simulink model "rate_limited_systems_controller_design"  (R2021a)
settings: Solver=VariableStepAuto  StartTime=0.0  StopTime=25  RelTol=1e-3
values from neighbouring files (symbols this model uses):
  K_P = 1/abs(freqresp(G_ol,omega_c))    [Anti_windup_example.m]    (also in P_Lead_Lag.m = 1/abs(freqresp(G_ol,omega_c*1i)); Rate_limited_example.m; Rate_limited_exercise.m)
undefined symbols (not defined in the file or in its folder): den_D, den_PI, num_D, num_PI
settings Model: Creator=dimpa  LastModifiedBy=dimpa

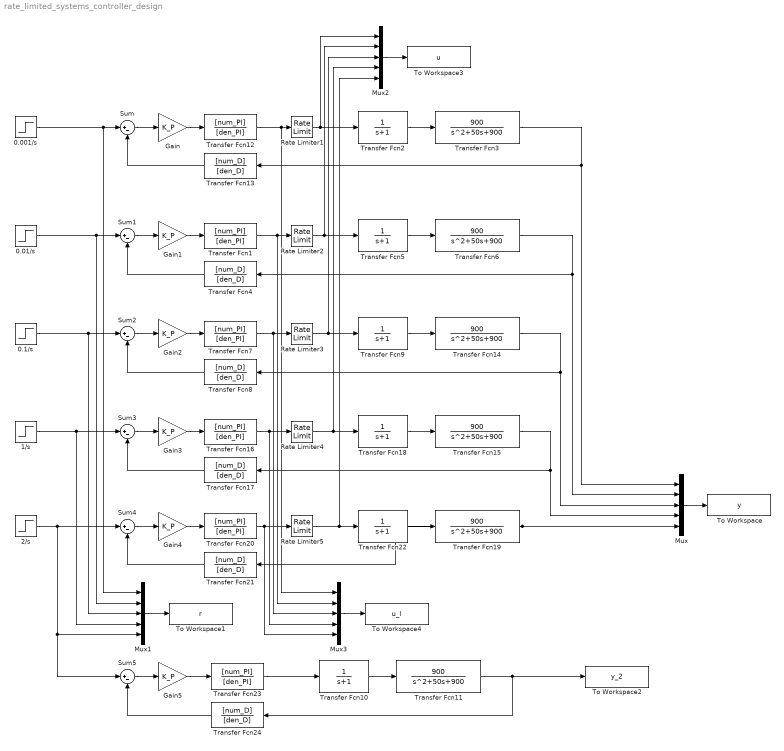
== system rate_limited_systems_controller_design ==
  0.001/s : Step  After=0.001  SampleTime=0
  0.01/s : Step  After=0.01  SampleTime=0
  0.1/s : Step  After=0.1  SampleTime=0
  1/s : Step  SampleTime=0
  2/s : Step  After=2  SampleTime=0
  Gain{,1..5} (6 alike) : Gain  Gain=K_P
  Mux{,1..3} (4 alike) : Mux  Inputs=5
  Rate Limiter{1..5} (5 alike) : RateLimiter  RisingSlewLimit=0.3  SampleTimeMode=inherited
  Sum{,1..5} (6 alike) : Sum  Inputs=|+-
  To Workspace : ToWorkspace  VariableName=y  SaveFormat=Timeseries  SampleTime=-1
  To Workspace1 : ToWorkspace  VariableName=r  SaveFormat=Timeseries  SampleTime=-1
  To Workspace2 : ToWorkspace  VariableName=y_2  SaveFormat=Timeseries  SampleTime=-1
  To Workspace3 : ToWorkspace  VariableName=u  SaveFormat=Timeseries  SampleTime=-1
  To Workspace4 : ToWorkspace  VariableName=u_l  SaveFormat=Timeseries  SampleTime=-1
  Transfer Fcn{1,7,12,16,20,23} (6 alike) : TransferFcn  Numerator=[num_PI]  Denominator=[den_PI]
  Transfer Fcn{2,5,9..10,18,22} (6 alike) : TransferFcn  Denominator=[1 1]
  Transfer Fcn{3,6,11,14..15,19} (6 alike) : TransferFcn  Numerator=[900]  Denominator=[1 50 900]
  Transfer Fcn{4,8,13,17,21,24} (6 alike) : TransferFcn  Numerator=[num_D]  Denominator=[den_D]
  wires:
  0.001/s/1 -> Sum/1, Mux1/1
  0.01/s/1 -> Sum1/1, Mux1/2
  0.1/s/1 -> Sum2/1, Mux1/3
  1/s/1 -> Sum3/1, Mux1/4
  2/s/1 -> Sum4/1, Sum5/1, Mux1/5
  Transfer Fcn19/1 -> Mux/5, Transfer Fcn21/1
  Transfer Fcn2/1 -> Transfer Fcn3/1
  Rate Limiter1/1 -> Transfer Fcn2/1, Mux2/1
  Transfer Fcn15/1 -> Transfer Fcn17/1, Mux/4
  Transfer Fcn14/1 -> Transfer Fcn8/1, Mux/3
  Transfer Fcn6/1 -> Transfer Fcn4/1, Mux/2
  Transfer Fcn3/1 -> Transfer Fcn13/1, Mux/1
  Mux/1 -> To Workspace/1
  Mux1/1 -> To Workspace1/1
  Transfer Fcn10/1 -> Transfer Fcn11/1
  Sum/1 -> Gain/1
  Gain/1 -> Transfer Fcn12/1
  Transfer Fcn12/1 -> Mux3/1, Rate Limiter1/1
  Transfer Fcn13/1 -> Sum/2
  Transfer Fcn4/1 -> Sum1/2
  Transfer Fcn1/1 -> Mux3/2, Rate Limiter2/1
  Gain1/1 -> Transfer Fcn1/1
  Sum1/1 -> Gain1/1
  Rate Limiter2/1 -> Transfer Fcn5/1, Mux2/2
  Transfer Fcn5/1 -> Transfer Fcn6/1
  Transfer Fcn9/1 -> Transfer Fcn14/1
  Rate Limiter3/1 -> Mux2/3, Transfer Fcn9/1
  Sum2/1 -> Gain2/1
  Gain2/1 -> Transfer Fcn7/1
  Transfer Fcn7/1 -> Mux3/3, Rate Limiter3/1
  Transfer Fcn8/1 -> Sum2/2
  Transfer Fcn17/1 -> Sum3/2
  Transfer Fcn16/1 -> Mux3/4, Rate Limiter4/1
  Gain3/1 -> Transfer Fcn16/1
  Sum3/1 -> Gain3/1
  Rate Limiter4/1 -> Mux2/4, Transfer Fcn18/1
  Transfer Fcn18/1 -> Transfer Fcn15/1
  Transfer Fcn22/1 -> Transfer Fcn19/1
  Rate Limiter5/1 -> Mux2/5, Transfer Fcn22/1
  Sum4/1 -> Gain4/1
  Gain4/1 -> Transfer Fcn20/1
  Transfer Fcn20/1 -> Mux3/5, Rate Limiter5/1
  Transfer Fcn21/1 -> Sum4/2
  Transfer Fcn24/1 -> Sum5/2
  Gain5/1 -> Transfer Fcn23/1
  Sum5/1 -> Gain5/1
  Transfer Fcn11/1 -> Transfer Fcn24/1, To Workspace2/1
  Transfer Fcn23/1 -> Transfer Fcn10/1
  Mux2/1 -> To Workspace3/1
  Mux3/1 -> To Workspace4/1
